simulink subsystem "tehrani_alv_mass_balance_v3"  (R2019b)
settings: Solver=VariableStepAuto  StartTime=0.0  StopTime=10.0  RelTol=1e-3
settings Model: Creator=RH  LastModifiedBy=RH

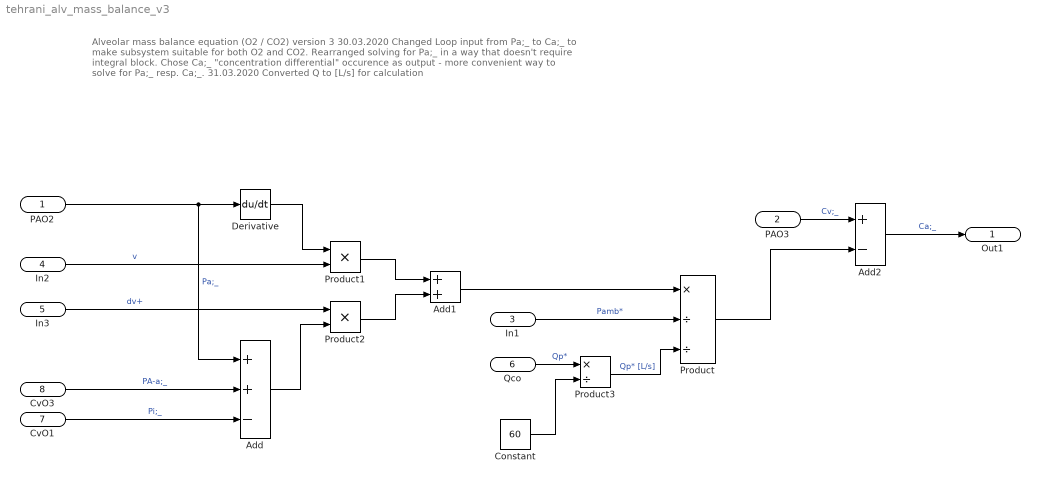
== system tehrani_alv_mass_balance_v3 ==
  note: Alveolar mass balance equation (O2 / CO2) version 3
      |
      | 30.03.2020 Changed Loop input from Pa;_ to Ca;_ to make subsystem suitable for both O2 and CO2.
      | Rearranged solving for Pa;_ in a way that doesn't require integral block.
      | Chose Ca;_ "concentration differential" occurence as output - more convenient way to solve for Pa;_ resp. Ca;_.
      | 31.03.2020 Converted Q to [L/s] for calculation
  PAO2 : Inport  Unit=mmHg
  PAO3 : Inport  Port=2  Unit=1
  In1 : Inport  Port=3  Unit=mmHg
  In2 : Inport  Port=4  Unit=L
  In3 : Inport  Port=5  Unit=L/s
  Qco : Inport  Port=6  Unit=L/min
  CvO1 : Inport  Port=7  Unit=mmHg
  CvO3 : Inport  Port=8  Unit=mmHg
  Add : Sum  Inputs=++-
  Add1 : Sum
  Add2 : Sum  Inputs=+-
  Constant : Constant  Value=60
  Derivative : Derivative
  Product : Product  Inputs=*//
  Product1 : Product
  Product2 : Product
  Product3 : Product  Inputs=*/
  Out1 : Outport  Unit=1
  wires:
  PAO2/1 -> Derivative/1, Add/1  "Pa;_"
  PAO3/1 -> Add2/1  "Cv;_"
  Qco/1 -> Product3/1  "Qp*"
  In1/1 -> Product/2  "Pamb*"
  In2/1 -> Product1/2  "v"
  Derivative/1 -> Product1/1
  In3/1 -> Product2/1  "dv+"
  Add/1 -> Product2/2
  CvO1/1 -> Add/3  "Pi;_"
  CvO3/1 -> Add/2  "PA-a;_"
  Product1/1 -> Add1/1
  Product2/1 -> Add1/2
  Add1/1 -> Product/1
  Product/1 -> Add2/2
  Add2/1 -> Out1/1  "Ca;_"
  Constant/1 -> Product3/2
  Product3/1 -> Product/3  "Qp* [L/s]"
